simulink model "EvitaParedes"  (R2023b)
settings: Solver=FixedStepAuto  StartTime=0.0  StopTime=inf  RelTol=1e-3  EnableMultiTasking=on
settings Model: ExtModeTrigDuration=2  Creator=Usuario_UMA  LastModifiedBy=Guerra
settings OptimizationCC: EnhancedBackFolding=on  PassReuseOutputArgsAs=Individual arguments  ZeroExternalMemoryAtStartup=off  ZeroInternalMemoryAtStartup=off  MaxStackSize=64  OptimizeBlockOrder=speed  DifferentSizesBufferReuse=on  OptimizationCustomize=off  EfficientTunableParamExpr=on
settings DebuggingCC: ParameterTunabilityLossMsg=error
settings HardwareCC: ProdBitPerInt=16  ProdBitPerPointer=16  ProdBitPerSizeT=16  ProdBitPerPtrDiffT=16  ProdLargestAtomicFloat=None  ProdWordSize=8  ProdHWDeviceType=Atmel->AVR
settings SFSimCC: MATLABDynamicMemAlloc=off
settings RTWCC: Description=Embedded Coder  SystemTargetFile=ert.tlc  HardwareBoard=Arduino Mega 2560  TemplateMakefile=ert_default_tmf  Toolchain=Arduino AVR  BuildConfiguration=Faster Runs
settings CodeAppCC: ForceParamTrailComments=on  IgnoreCustomStorageClasses=off  OperatorAnnotations=on  SimulinkDataObjDesc=on  SFDataObjDesc=on  InsertBlockDesc=on
settings ERTTargetCC: SupportContinuousTime=on  SupportVariableSizeSignals=on  ExtModeTransport=3  ExtModeStaticAlloc=on  ExtModeAutomaticAllocSize=off  ExtModeStaticAllocSize=2048  ExtModeMexFile=ext_xcp  ExtModeIntrfLevel=Level2 - Open

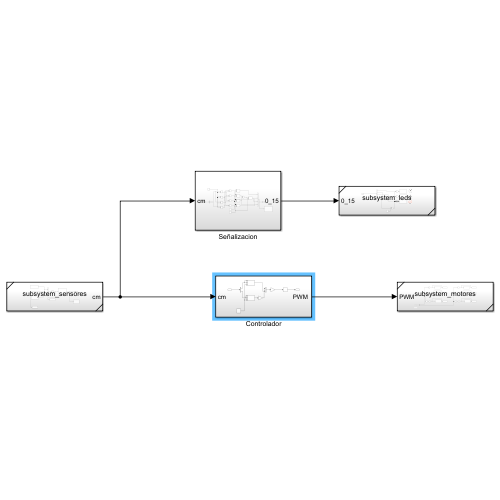
[thumbnail: Simulink's stored preview of the top-level diagram]
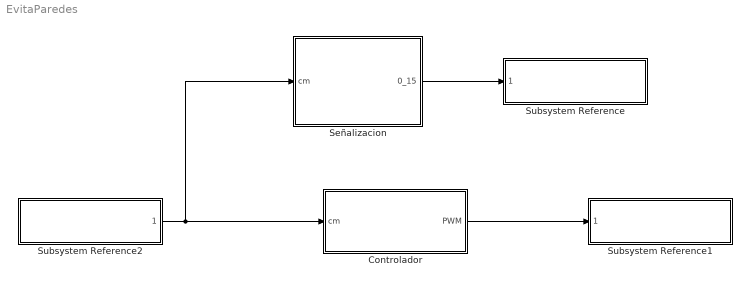
== system EvitaParedes ==
  Controlador : Subsystem
  Señalizacion : Subsystem
  Subsystem Reference : Subsystem  ReferencedSubsystem=subsystem_leds
  Subsystem Reference1 : Subsystem  ReferencedSubsystem=subsystem_motores
  Subsystem Reference2 : Subsystem  ReferencedSubsystem=subsystem_sensores
  wires:
  Subsystem Reference2/1 -> Controlador/1(cm), Señalizacion/1(cm)
  Controlador/1("PWM ") -> Subsystem Reference1/1
  Señalizacion/1(0_15) -> Subsystem Reference/1

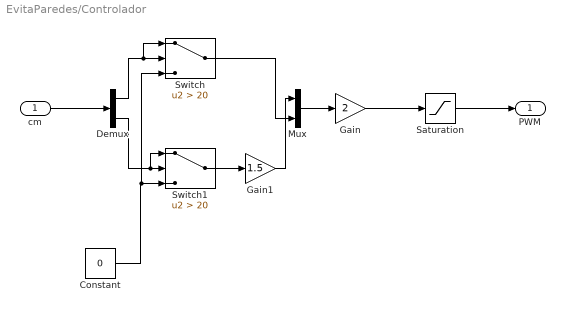
== system EvitaParedes/Controlador ==
  cm : Inport
  Constant : Constant  Value=0
  Demux : Demux  Outputs=2
  Gain : Gain  Gain=2
  Gain1 : Gain  Gain=1.5
  Mux : Mux  Inputs=2
  Saturation : Saturate  UpperLimit=30  LowerLimit=0
  Switch : Switch  Criteria=u2 > Threshold  Threshold=20  SaturateOnIntegerOverflow=off  InputSameDT=off
  Switch1 : Switch  Criteria=u2 > Threshold  Threshold=20  SaturateOnIntegerOverflow=off  InputSameDT=off
  "PWM " : Outport
  wires:
  Mux/1 -> Gain/1
  Saturation/1 -> "PWM "/1
  cm/1 -> Demux/1
  Gain/1 -> Saturation/1
  Constant/1 -> Switch/3, Switch1/3
  Demux/1 -> Switch/1, Switch/2
  Demux/2 -> Switch1/1, Switch1/2
  Switch/1 -> Mux/2
  Switch1/1 -> Gain1/1
  Gain1/1 -> Mux/1

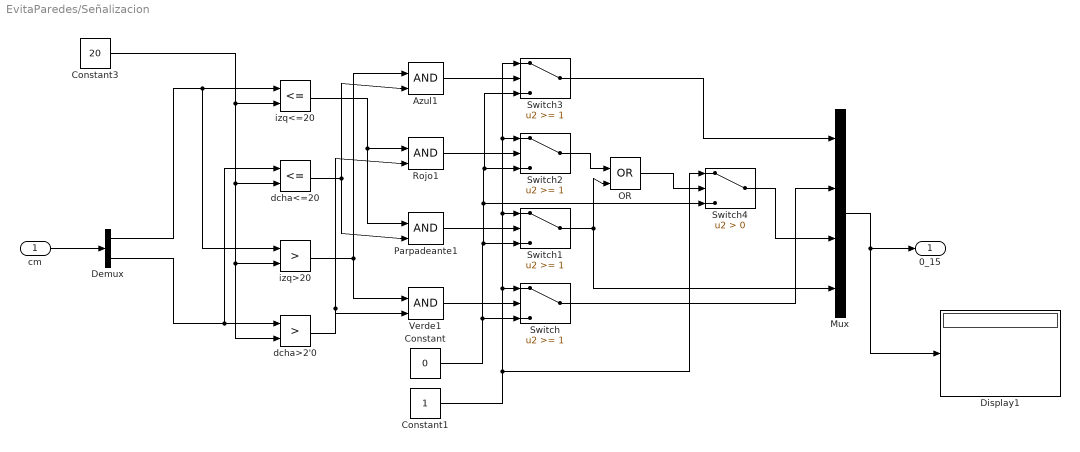
== system EvitaParedes/Señalizacion ==
  cm : Inport
  Azul1 : Logic  IconShape=distinctive  AllPortsSameDT=off  OutDataTypeStr=boolean
  Constant : Constant  Value=0
  Constant1 : Constant
  Constant3 : Constant  Value=20
  Demux : Demux  Outputs=2
  Display1 : Display
  Mux : Mux
  OR : Logic  Operator=OR  IconShape=distinctive  AllPortsSameDT=off  OutDataTypeStr=boolean
  Parpadeante1 : Logic  IconShape=distinctive  AllPortsSameDT=off  OutDataTypeStr=boolean
  Rojo1 : Logic  IconShape=distinctive  AllPortsSameDT=off  OutDataTypeStr=boolean
  Switch : Switch  Threshold=1  SaturateOnIntegerOverflow=off  InputSameDT=off
  Switch1 : Switch  Threshold=1  ZeroCross=off  SaturateOnIntegerOverflow=off  InputSameDT=off
  Switch2 : Switch  Threshold=1  SaturateOnIntegerOverflow=off  InputSameDT=off
  Switch3 : Switch  Threshold=1  SaturateOnIntegerOverflow=off  InputSameDT=off
  Switch4 : Switch  Criteria=u2 > Threshold  SaturateOnIntegerOverflow=off  InputSameDT=off
  Verde1 : Logic  IconShape=distinctive  AllPortsSameDT=off  OutDataTypeStr=boolean
  dcha<=20 : RelationalOperator  Operator=<=  OutDataTypeStr=boolean  RndMeth=Simplest  InputSameDT=off
  dcha>2'0 : RelationalOperator  Operator=>  OutDataTypeStr=boolean  RndMeth=Simplest  InputSameDT=off
  izq<=20 : RelationalOperator  Operator=<=  OutDataTypeStr=boolean  RndMeth=Simplest  InputSameDT=off
  izq>20 : RelationalOperator  Operator=>  OutDataTypeStr=boolean  RndMeth=Simplest  InputSameDT=off
  0_15 : Outport
  wires:
  Constant1/1 -> Switch4/1, Switch/1, Switch1/1, Switch2/1, Switch3/1
  Azul1/1 -> Switch3/2
  Parpadeante1/1 -> Switch1/2
  Switch1/1 -> OR/2, Mux/4
  Verde1/1 -> Switch/2
  Rojo1/1 -> Switch2/2
  dcha>2'0/1 -> Rojo1/2, Verde1/2
  dcha<=20/1 -> Parpadeante1/2, Azul1/2
  Constant3/1 -> dcha>2'0/2, izq>20/2, dcha<=20/2, izq<=20/2
  Mux/1 -> Display1/1, 0_15/1
  izq<=20/1 -> Rojo1/1, Parpadeante1/1
  izq>20/1 -> Verde1/1, Azul1/1
  Switch3/1 -> Mux/1
  Constant/1 -> Switch4/3, Switch3/3, Switch2/3, Switch1/3, Switch/3
  cm/1 -> Demux/1
  Demux/1 -> izq>20/1, izq<=20/1
  Demux/2 -> dcha<=20/1, dcha>2'0/1
  Switch2/1 -> OR/1
  OR/1 -> Switch4/2
  Switch/1 -> Mux/2
  Switch4/1 -> Mux/3
